simulink model "TIVA123n_adc_16b"  (R2016b)
settings: Solver=ode3  StartTime=0.0  StopTime=inf  RelTol=1e-3  EnableMultiTasking=on
libraries: energialib x4, dspstat3 x2
settings Model: SimulationMode=external  ExtModeTrigDuration=10  Creator=ppashine  LastModifiedBy=marto
settings DataIOCC: Decimation=3  LimitDataPoints=on  MaxDataPoints=10000  SaveFormat=Array  InspectSignalLogs=on  LoggingToFile=on
settings OptimizationCC: LifeSpan=1  MaxStackSize=64
settings DebuggingCC: AllowSymbolicDim=off  SFUnexpectedBacktrackingDiag=warning  SFNoUnconditionalDefaultTransitionDiag=warning  SFExecutionAtInitializationDiag=none
settings HardwareCC: ProdBitPerPointer=32  ProdBitPerSizeT=32  ProdBitPerPtrDiffT=32  ProdLargestAtomicInteger=Long  ProdLargestAtomicFloat=Double  ProdWordSize=32  ProdHWDeviceType=ARM Compatible->ARM Cortex
settings ModelReferenceCC: PropagateSignalLabelsOutOfModel=off
settings RTWCC: SystemTargetFile=ert.tlc  HardwareBoard=Tiva TM4C123G LaunchPad  TLCOptions=-aInlineSetEventsForThisBaseRateFcn=TLC_FALSE -aSuppressMultiTaskScheduler=TLC_FALSE -aRateBasedStepFcn=1  TemplateMakefile=ert_default_tmf  Description=Embedded Coder  Toolchain=Energia Tiva  BuildConfiguration=Faster Runs
settings CodeAppCC: IgnoreCustomStorageClasses=off
settings ERTTargetCC: ConvertIfToSwitch=off  SuppressUnreachableDefaultCases=off
settings ConfigComp: CovMetricSettings=dw  CovHtmlReporting=on  CovSaveCumulativeToWorkspaceVar=on  CovSaveSingleToWorkspaceVar=on  CovExternalEMLEnable=off

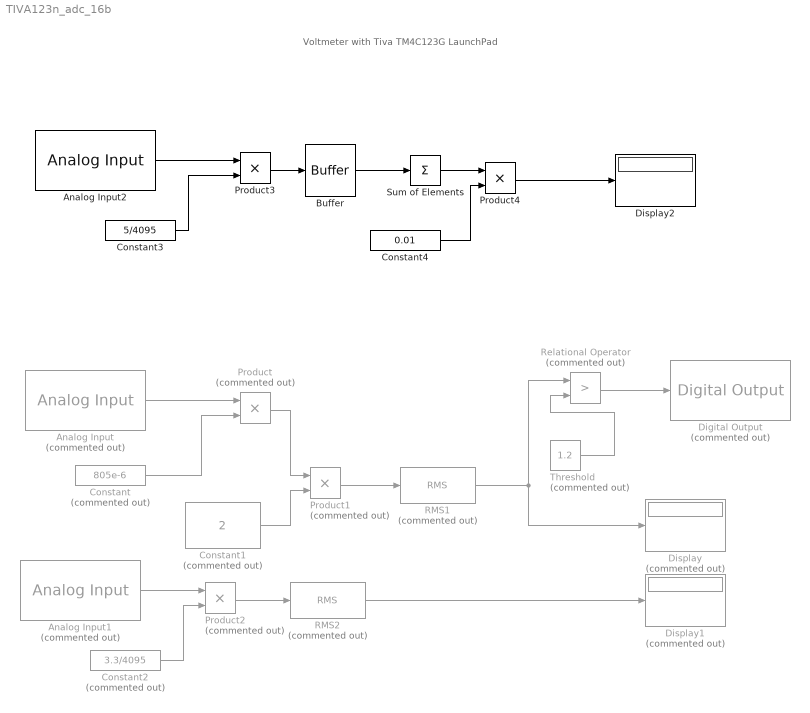
== system TIVA123n_adc_16b ==
  note: Voltmeter with Tiva TM4C123G LaunchPad
  Analog Input : energialib/Analog Input  Commented=on  pinNumber=7  sampleTime=0.001  blockPlatform=energia
  Analog Input1 : energialib/Analog Input  Commented=on  pinNumber=23  sampleTime=0.001  blockPlatform=energia
  Analog Input2 : energialib/Analog Input  pinNumber=24  sampleTime=0.001  blockPlatform=energia
  Buffer : Buffer  N=100  TreatMby1Signals=One channel  OutputFrames=off
  Constant : Constant  Commented=on  Value=805e-6  SampleTime=0.001
  Constant1 : Constant  Commented=on  Value=2  SampleTime=0.001
  Constant2 : Constant  Commented=on  Value=3.3/4095  SampleTime=0.001
  Constant3 : Constant  Value=5/4095  SampleTime=0.001
  Constant4 : Constant  Value=0.01  SampleTime=0.1
  Digital Output : energialib/Digital Output  Commented=on  pinNumber=39  blockPlatform=energia
  Display : Display  Commented=on
      settings: Decimation=3
  Display1 : Display  Commented=on
      settings: Decimation=3
  Display2 : Display
      settings: Decimation=3
  Product : Product  Commented=on
  Product1 : Product  Commented=on
  Product2 : Product  Commented=on
  Product3 : Product
  Product4 : Product
  RMS1 : dspstat3/RMS  Commented=on  run=off  directionMode=Each column  dimension=100  reset_popup=None
  RMS2 : dspstat3/RMS  Commented=on  run=off  directionMode=Each column  dimension=100  reset_popup=None
  Relational Operator : RelationalOperator  Commented=on  Operator=>  OutDataTypeStr=fixdt(1,16)  RndMeth=Nearest
  Sum of Elements : Sum  Inputs=+
  "Threshold " : Constant  Commented=on  Value=1.2  OutDataTypeStr=uint8  SampleTime=0.001
  wires:
  Analog Input/1 -> Product/1
  "Threshold "/1 -> Relational Operator/2
  Relational Operator/1 -> Digital Output/1
  RMS1/1 -> Relational Operator/1, Display/1
  Constant/1 -> Product/2
  Product/1 -> Product1/1
  Product1/1 -> RMS1/1
  Constant1/1 -> Product1/2
  Analog Input1/1 -> Product2/1
  Constant2/1 -> Product2/2
  Product2/1 -> RMS2/1
  RMS2/1 -> Display1/1
  Product3/1 -> Buffer/1
  Analog Input2/1 -> Product3/1
  Constant3/1 -> Product3/2
  Buffer/1 -> Sum of Elements/1
  Sum of Elements/1 -> Product4/1
  Product4/1 -> Display2/1
  Constant4/1 -> Product4/2
